simulink model "Stepper_Model_2017_10_31"  (R2017a)
settings: Solver=VariableStepAuto  StartTime=0.0  StopTime=tsim  RelTol=1e-3
model workspace (MAT data in the model file):
  V = Simulink.Signal
  V.DataType = 'auto'
  V.Dimensions = -1
  V.DimensionsMode = 'auto'
  V.Complexity = 'auto'
  V.SampleTime = -1
  V.SamplingMode = 'auto'
values from neighbouring files (symbols this model uses):
  c = 0.05    [Stepper_Model_2017_10_31_Script.m]    (also in pendcartsim.m)
  Controller_Gain = -3.5    [Stepper_Model_2017_10_31_Script.m]
  g = 9.82    [Stepper_Model_2017_10_31_Script.m]    (also in pendcartsim.m)
  K2 = 1.402    [Stepper_Model_2017_10_31_Script.m]    (also in pendcartsim.m = 0.0402)
  L = 0.8    [Stepper_Model_2017_10_31_Script.m]
  m = 0.25    [Stepper_Model_2017_10_31_Script.m]    (also in pendcartsim.m = 0.5)
  M = 1    [Stepper_Model_2017_10_31_Script.m]    (also in pendcartsim.m)
  poles = 2.2    [Stepper_Model_2017_10_31_Script.m]
  wheel_Radius = 0.088    [Stepper_Model_2017_10_31_Script.m]
  zeroes = 1    [Stepper_Model_2017_10_31_Script.m]
undefined symbols (not defined in the file or in its folder): sigbuilder_block
settings Model: Creator=Administrator  LastModifiedBy=Administrator

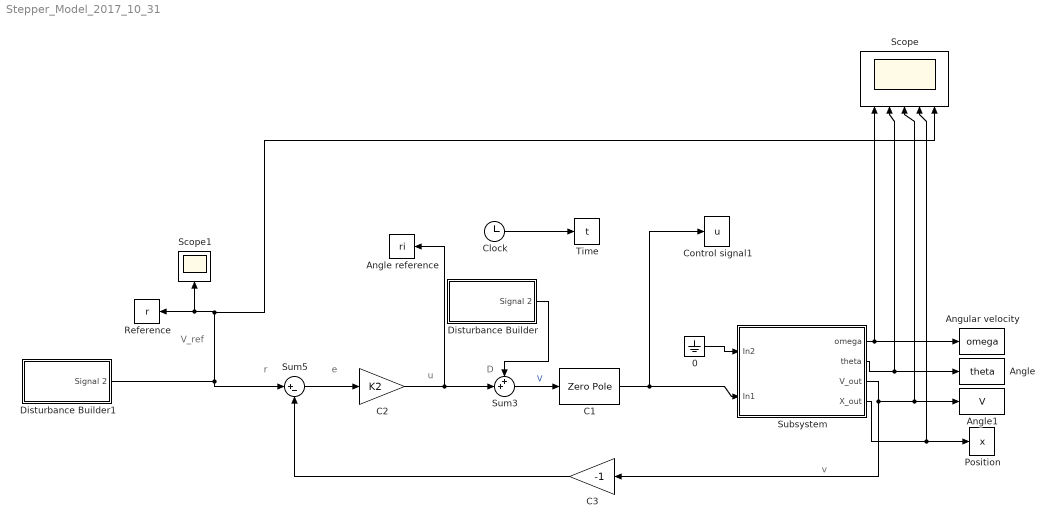
== system Stepper_Model_2017_10_31 ==
  note: V_ref
  note: D
  note: v
  note: u
  note: e
  note: r
  0 : Ground
  Angle : ToWorkspace  VariableName=theta  SampleTime=-1
  Angle reference : ToWorkspace  VariableName=ri  SampleTime=-1
  Angle1 : ToWorkspace  VariableName=V  SampleTime=-1
  Angular velocity : ToWorkspace  VariableName=omega  SampleTime=-1
  C1 : ZeroPole  Zeros=[-zeroes]  Poles=[-poles]  Gain=[Controller_Gain]  ContinuousStateAttributes='Velocity'
  C2 : Gain  Gain=K2
  C3 : Gain  Gain=-1
  Clock : Clock
  Control signal1 : ToWorkspace  VariableName=u  SampleTime=-1
  Disturbance Builder : Subsystem  Tag=STV Subsys  LoadFcn=sigbuilder_block('load');  StartFcn=sigbuilder_block('start');  StopFcn=sigbuilder_block('stop');  ClipboardFcn=sigbuilder_block('clipboard');  mask(Sigbuilder block){tuvar=[0:10]}
      mask help: Simulink:masks:SigbuilderBlock_MD
      mask init:
      | if ~strcmp(get_param(bdroot(gcbh),'SimulationStatus'),'stopped') tuvar = sigbuilder_block('maskInit'); end
      settings: CopyFcn=sigbuilder_block('copy');  DeleteFcn=sigbuilder_block('delete');  ModelCloseFcn=sigbuilder_block('modelClose');  PreSaveFcn=sigbuilder_block('preSave');  PauseFcn=sigbuilder_block('pause');  ContinueFcn=sigbuilder_block('continue');  NameChangeFcn=sigbuilder_block('namechange');  OpenFcn=sigbuilder_block('open',[203 87.5 550.5 362.5 ]);  CloseFcn=sigbuilder_block('close');
      mask Display: plot(0, 0, 100, 100,[2, 2, 32, 32, 2], [68, 8, 8, 68, 68],[32, 2], [38, 38], [32, 19, 2],[53, 60, 44], [32, 17, 17, 2],[16, 16, 31, 31]);txt = getActiveGroup(gcbh);text(2, 100, txt,'verticalAlignment', 'top');
  Disturbance Builder1 : Subsystem  Tag=STV Subsys  LoadFcn=sigbuilder_block('load');  StartFcn=sigbuilder_block('start');  StopFcn=sigbuilder_block('stop');  ClipboardFcn=sigbuilder_block('clipboard');  mask(Sigbuilder block){tuvar=[0:10]}
      mask help: Simulink:masks:SigbuilderBlock_MD
      mask init:
      | if ~strcmp(get_param(bdroot(gcbh),'SimulationStatus'),'stopped') tuvar = sigbuilder_block('maskInit'); end
      settings: CopyFcn=sigbuilder_block('copy');  DeleteFcn=sigbuilder_block('delete');  ModelCloseFcn=sigbuilder_block('modelClose');  PreSaveFcn=sigbuilder_block('preSave');  PauseFcn=sigbuilder_block('pause');  ContinueFcn=sigbuilder_block('continue');  NameChangeFcn=sigbuilder_block('namechange');  OpenFcn=sigbuilder_block('open',[203 87.5 550.5 362.5 ]);  CloseFcn=sigbuilder_block('close');
      mask Display: plot(0, 0, 100, 100,[2, 2, 32, 32, 2], [68, 8, 8, 68, 68],[32, 2], [38, 38], [32, 19, 2],[53, 60, 44], [32, 17, 17, 2],[16, 16, 31, 31]);txt = getActiveGroup(gcbh);text(2, 100, txt,'verticalAlignment', 'top');
  Position : ToWorkspace  VariableName=x  SampleTime=-1
  Reference : ToWorkspace  VariableName=r  SampleTime=-1
  Scope : Scope  NumInputPorts=5
  Scope1 : Scope
  Subsystem : Subsystem
  Sum3 : Sum  Inputs=++|
  Sum5 : Sum  Inputs=|+-
  Time : ToWorkspace  VariableName=t  SampleTime=-1
  wires:
  0/1 -> Subsystem/1(In2)
  C2/1 -> Sum3/2, Angle reference/1
  Sum5/1 -> C2/1
  Subsystem/2(theta) -> Scope/2, Angle/1
  Sum3/1 -> C1/1  "V"
  Clock/1 -> Time/1
  Disturbance Builder1/1(Signal 2) -> Sum5/1, Scope/5, Scope1/1, Reference/1
  Disturbance Builder/1(Signal 2) -> Sum3/1
  C3/1 -> Sum5/2
  Subsystem/1(omega) -> Angular velocity/1, Scope/1
  Subsystem/3(V_out) -> C3/1, Scope/3, Angle1/1
  Subsystem/4(X_out) -> Position/1, Scope/4
  C1/1 -> Subsystem/2(In1), Control signal1/1

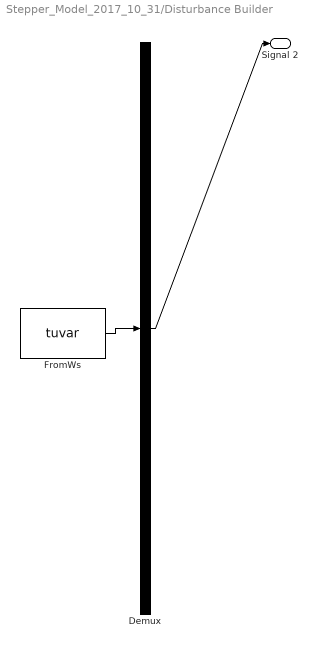
== system Stepper_Model_2017_10_31/Disturbance Builder ==
  Demux : Demux  Tag=STV Demux  Outputs=1
  FromWs : FromWorkspace  Tag=STV FromWs  VariableName=tuvar  SampleTime=0
      SigBuilderData=|
      | common.afterFinalStr = 'Extrapolate'
      | common.sampleTime = 0
      | dataSet.timeRange = [0 10]
      | dataSet.name = 'Group 1'
      | sbobj.Groups.Name = 'Group 1'
      | sbobj.Groups.Signals.Name = 'Signal 2'
      | sbobj.Groups.Signals.XData = [0 10]
      | sbobj.Groups.Signals.YData = [0 0]
  Signal 2 : Outport  Tag=STV Outport
  wires:
  FromWs/1 -> Demux/1
  Demux/1 -> Signal 2/1

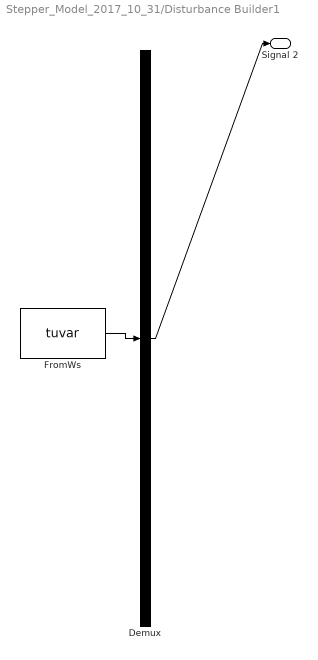
== system Stepper_Model_2017_10_31/Disturbance Builder1 ==
  Demux : Demux  Tag=STV Demux  Outputs=1
  FromWs : FromWorkspace  Tag=STV FromWs  VariableName=tuvar  SampleTime=0
      SigBuilderData=|
      | common.afterFinalStr = 'Extrapolate'
      | common.sampleTime = 0
      | dataSet.timeRange = [0 10]
      | dataSet.name = 'Group 1'
      | sbobj.Groups.Name = 'Group 1'
      | sbobj.Groups.Signals.Name = 'Signal 2'
      | sbobj.Groups.Signals.XData = [0 10]
      | sbobj.Groups.Signals.YData = [0 0]
  Signal 2 : Outport  Tag=STV Outport
  wires:
  FromWs/1 -> Demux/1
  Demux/1 -> Signal 2/1

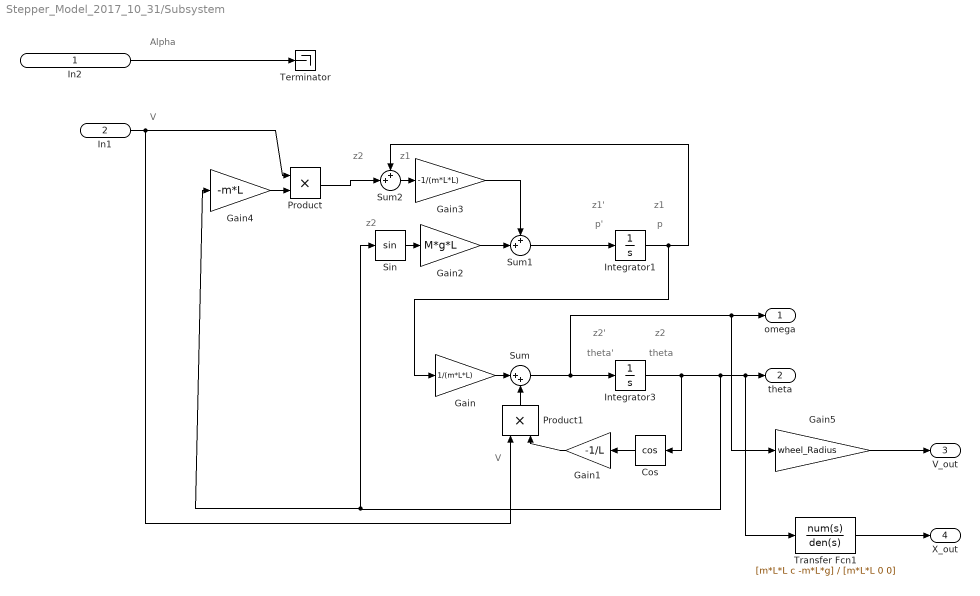
== system Stepper_Model_2017_10_31/Subsystem ==
  note: V
  note: V
  note: z2
  note: z2
  note: z2'
  note: z1
  note: z1'
  note: theta
  note: p
  note: theta'
  note: p'
  note: z2
  note: z1
  note: Alpha
  In2 : Inport
  In1 : Inport  Port=2
  Cos : Trigonometry  Operator=cos
  Gain : Gain  Gain=1/(m*L*L)
  Gain1 : Gain  Gain=-1/L
  Gain2 : Gain  Gain=M*g*L
  Gain3 : Gain  Gain=-1/(m*L*L)
  Gain4 : Gain  Gain=-m*L
  Gain5 : Gain  Gain=wheel_Radius
  Integrator1 : Integrator
  Integrator3 : Integrator
  Product : Product
  Product1 : Product
  Sin : Trigonometry
  Sum : Sum  Inputs=|++
  Sum1 : Sum  Inputs=++|
  Sum2 : Sum  Inputs=++|
  Terminator : Terminator
  Transfer Fcn1 : TransferFcn  Numerator=[m*L*L c -m*L*g]  Denominator=[m*L*L 0 0]  ContinuousStateAttributes='x'
  omega : Outport
  theta : Outport  Port=2
  V_out : Outport  Port=3
  X_out : Outport  Port=4
  wires:
  Sum1/1 -> Integrator1/1
  Gain4/1 -> Product/2
  Cos/1 -> Gain1/1
  Sin/1 -> Gain2/1
  In1/1 -> Product1/1, Product/1
  Sum2/1 -> Gain3/1
  Gain3/1 -> Sum1/1
  Gain2/1 -> Sum1/2
  Product/1 -> Sum2/2
  Integrator1/1 -> Sum2/1, Gain/1
  Integrator3/1 -> Transfer Fcn1/1, theta/1, Gain4/1, Sin/1, Cos/1
  Sum/1 -> Gain5/1, omega/1, Integrator3/1
  Gain/1 -> Sum/1
  In2/1 -> Terminator/1
  Gain5/1 -> V_out/1
  Transfer Fcn1/1 -> X_out/1
  Gain1/1 -> Product1/2
  Product1/1 -> Sum/2
